simulink model "manipulator_simulation"  (R2021a)
settings: Solver=VariableStepAuto  StartTime=0.0  StopTime=14  MaxStep=0.01  RelTol=1e-3
settings Model: Creator=bikra  LastModifiedBy=bikra
settings DebuggingCC: UnconnectedInputMsg=none  UnconnectedOutputMsg=none  UnconnectedLineMsg=none
settings RTWCC: DLArmComputeVersion=20.02.1

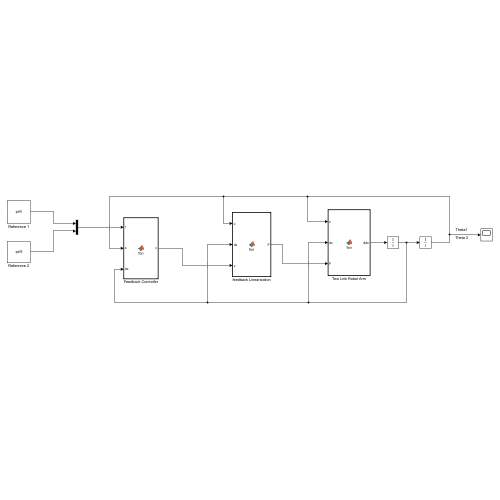
[thumbnail: Simulink's stored preview of the top-level diagram]
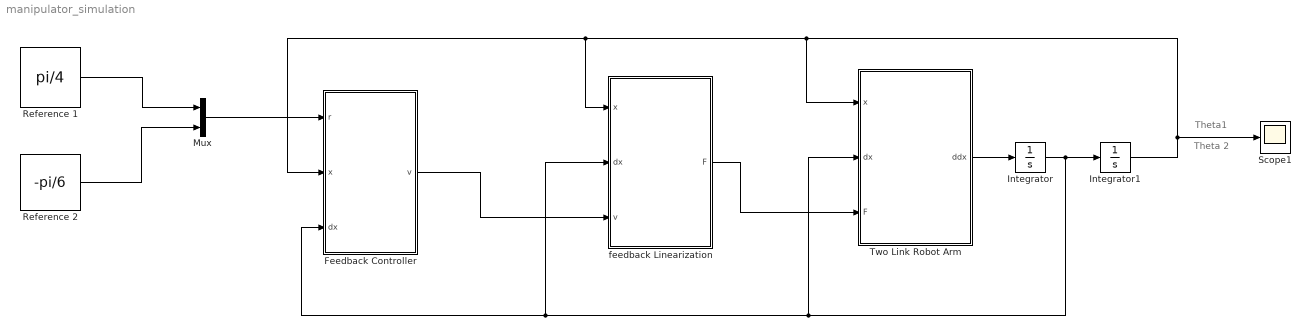
== system manipulator_simulation ==
  note: Theta 2
  note: Theta1
  Feedback Controller : MATLAB Function  TreatAsAtomicUnit=on
  Integrator : Integrator  InitialCondition=[0 0]
  Integrator1 : Integrator  InitialCondition=[pi/2 pi/2]
  Mux : Mux  Inputs=2
  Reference 1 : Constant  Value=pi/4
  Reference 2 : Constant  Value=-pi/6
  Scope1 : Scope
  Two Link Robot Arm : MATLAB Function  TreatAsAtomicUnit=on
  feedback Linearization : MATLAB Function  TreatAsAtomicUnit=on
  wires:
  Reference 1/1 -> Mux/1
  Reference 2/1 -> Mux/2
  Two Link Robot Arm/1(ddx) -> Integrator/1
  Integrator1/1 -> feedback Linearization/1(x), Feedback Controller/2(x), Two Link Robot Arm/1(x), Scope1/1
  Mux/1 -> Feedback Controller/1(r)
  Feedback Controller/1(v) -> feedback Linearization/3(v)
  Integrator/1 -> Integrator1/1, Feedback Controller/3(dx), feedback Linearization/2(dx), Two Link Robot Arm/2(dx)
  feedback Linearization/1(F) -> Two Link Robot Arm/3(F)

== matlab function manipulator_simulation/Two Link Robot Arm ==
  data: x input; dx input; F input; ddx output
function ddx = fcn(x,dx,F)

M1 = 1;
M2 = 1;
L1 = 2;
L2 = 1;
g = 9.81;
G = [-(M1+M2)*g*L1-M2*g*L2*sin(x(1)+x(2));
    -M2*g*L2*sin(x(1)+x(2));];
C = [M1*L1*L2*(2*dx(1)*dx(2) + dx(1)^2)*sin(x(2));
    -M2*L1*L2*dx(1)*dx(2)*sin(x(2));];
M = [-(M1+M2)*L1^2 + M2*L2^2 + 2*M2*L1*L2*cos(x(2)),    M2*L2^2 + M2*L1*L2*cos(x(2));
     M2*L2^2 + M2*L1*L2*cos(x(2)),  M2*L2^2;];
ddx = inv(M)*(-C-G+F);

== matlab function manipulator_simulation/Feedback Controller ==
  data: r input; v output; x input; dx input
function v  = fcn(r,x,dx)

k1 = 15.99;
k2 = 5.65;
k3 = k1;

v = [k3*r(1) - k1*x(1) - k2*dx(1);
     (k3*r(2) - k1*x(2) - k2*dx(2))];

== matlab function manipulator_simulation/feedback Linearization ==
  data: x input; dx input; F output; v input
function F = fcn(x,dx,v)

M1 = 1;
M2 = 1;
L1 = 2;
L2 = 1;
g = 9.81;
G = [-(M1+M2)*g*L1-M2*g*L2*sin(x(1)+x(2));...
    -M2*g*L2*sin(x(1)+x(2));];
C = [M1*L1*L2*(2*dx(1)*dx(2) + dx(1)^2)*sin(x(2));...
    -M2*L1*L2*dx(1)*dx(2)*sin(x(2));];
M = [-(M1+M2)*L1^2 + M2*L2^2 + 2*M2*L1*L2*cos(x(2)), M2*L2^2 + M2*L1*L2*cos(x(2));...
     M2*L2^2 + M2*L1*L2*cos(x(2)),  M2*L2^2;];



F = M*v + C + G;
